simulink model "cradle"  (R2013a)
settings: Solver=ode45  StartTime=0.0  StopTime=10.0  RelTol=1e-3
libraries: vrlib x6
settings Model: Creator=nilesh  LastModifiedBy=nilesh

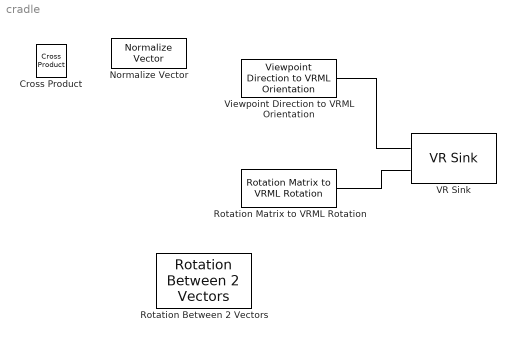
== system cradle ==
  Cross Product : vrlib/Utilities/Cross Product
  Normalize Vector : vrlib/Utilities/Normalize Vector  maxzero=0
  Rotation Between 2 Vectors : vrlib/Utilities/Rotation Between 2 Vectors
  Rotation Matrix to VRML Rotation : vrlib/Utilities/Rotation Matrix to VRML Rotation  maxzero=1e-12
  VR Sink : vrlib/VR Sink  InstantiateOnLoad=on  SampleTime=0.1  ViewEnable=on  RemoteChange=off  RemoteView=on  AutoView=off  VideoDimensions=[]  AllowVariableSize=off
  Viewpoint Direction to VRML Orientation : vrlib/Utilities/Viewpoint Direction to VRML Orientation
  wires:
  Viewpoint Direction to VRML Orientation/1 -> ?
  Rotation Matrix to VRML Rotation/1 -> ?
